simulink model "hamulec"  (R2018b)
settings: Solver=ode4  StartTime=0.0  StopTime=10  RelTol=1e-3
values from neighbouring files (symbols this model uses):
  g = 9.81    [dane.m]    (also in untitled.m)
  J_w = 0.01    [dane.m]    (also in untitled.m)
  m_v = 1200    [dane.m]
  r_w = 0.3    [dane.m]    (also in untitled.m)
settings Model: Creator=lpa1  LastModifiedBy=lpa1

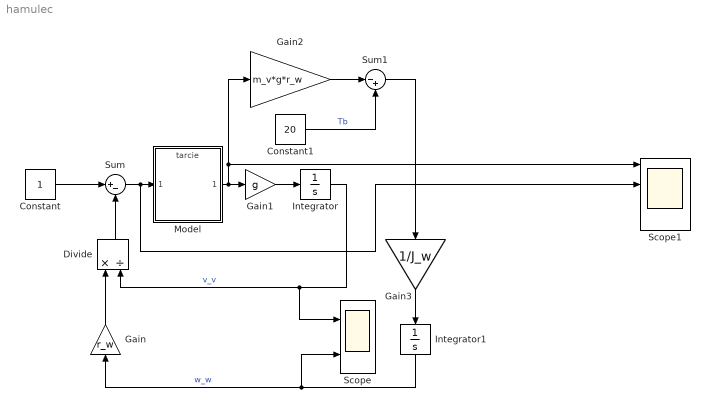
== system hamulec ==
  Constant : Constant
  Constant1 : Constant  Value=20
  Divide : Product  Inputs=*/
  Gain : Gain  Gain=r_w
  Gain1 : Gain  Gain=g
  Gain2 : Gain  Gain=m_v*g*r_w
  Gain3 : Gain  Gain=1/J_w
  Integrator : Integrator  InitialCondition=10
  Integrator1 : Integrator  InitialCondition=5
  Model : ModelReference  ModelNameDialog=tarcie.slx  SimulationMode=Normal  ModelReferenceVersion=1.10  SimulationMode=Normal
  Scope : Scope  NumInputPorts=2
  Scope1 : Scope  NumInputPorts=4
  Sum : Sum  Inputs=|+-
  Sum1 : Sum  Inputs=|-+
  wires:
  Constant/1 -> Sum/1
  Divide/1 -> Sum/2
  Sum/1 -> Scope1/2, Model/1
  Gain/1 -> Divide/1
  Model/1 -> Gain2/1, Scope1/1, Gain1/1
  Gain1/1 -> Integrator/1
  Integrator/1 -> Divide/2, Scope/1  "v_v"
  Sum1/1 -> Gain3/1
  Gain3/1 -> Integrator1/1
  Constant1/1 -> Sum1/2  "Tb"
  Gain2/1 -> Sum1/1
  Integrator1/1 -> Gain/1, Scope/2  "w_w"
